simulink model "Prac1_SimDPP"  (R2023b)
settings: Solver=ode23  StartTime=0.0  StopTime=200  RelTol=1e-3
values from neighbouring files (symbols this model uses):
  g = 9.81    [Prac1_SimDPP.mat]
  l1 = 0.3    [Prac1_SimDPP.mat]
  l2 = 0.25    [Prac1_SimDPP.mat]
  m1 = 0.2    [Prac1_SimDPP.mat]
  m2 = 0.1    [Prac1_SimDPP.mat]

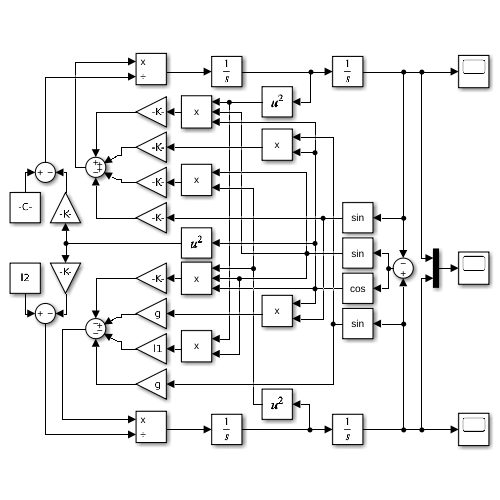
[thumbnail: Simulink's stored preview of the top-level diagram]
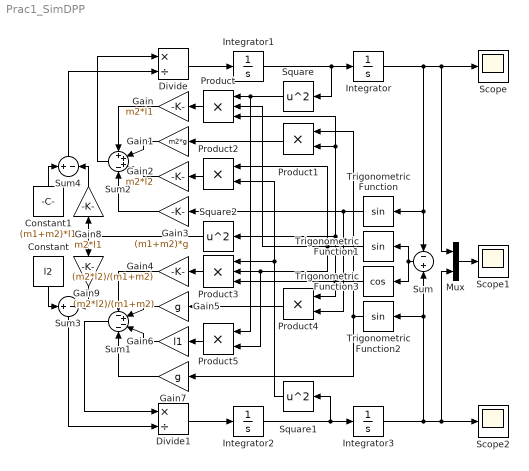
== system Prac1_SimDPP ==
  Constant : Constant  Value=l2
  Constant1 : Constant  Value=(m1+m2)*l1
  Divide : Product  Inputs=*/
  Divide1 : Product  Inputs=*/
  Gain : Gain  Gain=m2*l1
  Gain1 : Gain  Gain=m2*g
  Gain2 : Gain  Gain=m2*l2
  Gain3 : Gain  Gain=(m1+m2)*g
  Gain4 : Gain  Gain=(m2*l2)/(m1+m2)
  Gain5 : Gain  Gain=g
  Gain6 : Gain  Gain=l1
  Gain7 : Gain  Gain=g
  Gain8 : Gain  Gain=m2*l1
  Gain9 : Gain  Gain=(m2*l2)/(m1+m2)
  Integrator : Integrator
  Integrator1 : Integrator
  Integrator2 : Integrator
  Integrator3 : Integrator  InitialCondition=0.610865
  Mux : Mux  Inputs=2
  Product : Product  Inputs=3
  Product{1..2,4..5} (4 alike) : Product
  Product3 : Product  Inputs=3
  Scope : Scope
  Scope1 : Scope
  Scope2 : Scope
  Square : Math  Operator=square
  Square1 : Math  Operator=square
  Square2 : Math  Operator=square
  Sum : Sum  Inputs=-+
  Sum1 : Sum  Inputs=-+--
  Sum2 : Sum  Inputs=+++-
  Sum3 : Sum  Inputs=+-
  Sum4 : Sum  Inputs=+-
  Trigonometric Function : Trigonometry
  Trigonometric Function1 : Trigonometry
  Trigonometric Function2 : Trigonometry
  Trigonometric Function3 : Trigonometry  Operator=cos
  wires:
  Mux/1 -> Scope1/1
  Sum/1 -> Trigonometric Function3/1, Trigonometric Function1/1
  Integrator/1 -> Scope/1, Mux/1, Sum/1, Trigonometric Function/1
  Integrator2/1 -> Square1/1, Integrator3/1
  Integrator1/1 -> Square/1, Integrator/1
  Integrator3/1 -> Scope2/1, Mux/2, Sum/2, Trigonometric Function2/1
  Square/1 -> Product5/1, Product/1
  Trigonometric Function1/1 -> Product5/2, Product3/2, Product/2, Product2/1
  Trigonometric Function3/1 -> Product4/1, Product3/3, Square2/1, Product1/2, Product/3
  Product/1 -> Gain/1
  Trigonometric Function2/1 -> Gain7/1, Product1/1
  Product1/1 -> Gain1/1
  Product2/1 -> Gain2/1
  Square1/1 -> Product3/1, Product2/2
  Trigonometric Function/1 -> Product4/2, Gain3/1
  Gain/1 -> Sum2/1
  Gain1/1 -> Sum2/2
  Gain2/1 -> Sum2/3
  Gain3/1 -> Sum2/4
  Product3/1 -> Gain4/1
  Product4/1 -> Gain5/1
  Product5/1 -> Gain6/1
  Gain4/1 -> Sum1/1
  Gain6/1 -> Sum1/3
  Gain7/1 -> Sum1/4
  Square2/1 -> Gain9/1, Gain8/1
  Gain9/1 -> Sum3/2
  Gain8/1 -> Sum4/2
  Constant/1 -> Sum3/1
  Constant1/1 -> Sum4/1
  Sum2/1 -> Divide/1
  Divide1/1 -> Integrator2/1
  Divide/1 -> Integrator1/1
  Sum1/1 -> Divide1/1
  Sum4/1 -> Divide/2
  Sum3/1 -> Divide1/2
  Gain5/1 -> Sum1/2
